simulink model "ex2_lab1"  (Simulink 6.0)
settings: Solver=ode45  StartTime=0.0  StopTime=10.0  RelTol=1e-3
settings Model: LastModifiedBy=student

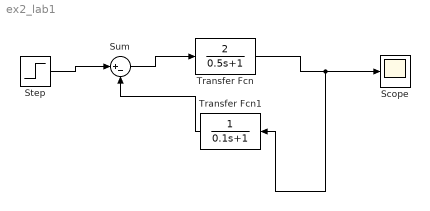
== system ex2_lab1 ==
  Scope : Scope
      settings: TimeRange=10  YMin=0  YMax=0.7000000000000001
  Step : Step  SampleTime=0
  Sum : Sum  Inputs=|+-
  Transfer Fcn : TransferFcn  Numerator=[2]  Denominator=[0.5 1]
  Transfer Fcn1 : TransferFcn  Orientation=left  Denominator=[0.1 1]
  wires:
  Transfer Fcn/1 -> Scope/1, Transfer Fcn1/1
  Step/1 -> Sum/1
  Sum/1 -> Transfer Fcn/1
  Transfer Fcn1/1 -> Sum/2
